simulink library "Hot_Water_Energy_Profile"  (R2018b)
settings: Solver=ode45  StartTime=0.0  StopTime=10.0  RelTol=1e-3  EnableMultiTasking=on
libraries: carnot x4
settings Model: Creator=lena.frank  LastModifiedBy=P41573
settings DataIOCC: LimitDataPoints=on  SaveFormat=Array  SignalLoggingSaveFormat=ModelDataLogs
settings OptimizationCC: ExpressionDepthLimit=2147483647  LifeSpan=inf
settings DebuggingCC: UnderspecifiedInitializationDetection=Classic  MergeDetectMultiDrivingBlocksExec=none  SolverPrmCheckMsg=warning  FcnCallInpInsideContextMsg=warning  StateNameClashWarn=warning  SFUnexpectedBacktrackingDiag=warning  SFNoUnconditionalDefaultTransitionDiag=warning  SFExecutionAtInitializationDiag=none
settings HardwareCC: ProdBitPerPointer=32  ProdBitPerSizeT=32  ProdBitPerPtrDiffT=32  ProdLargestAtomicFloat=None  ProdIntDivRoundTo=Undefined  ProdEndianess=Unspecified  ProdWordSize=32  ProdHWDeviceType=32-bit Generic
settings ModelReferenceCC: PropagateSignalLabelsOutOfModel=off
settings SFSimCC: SimUseLocalCustomCode=off
settings RTWCC: RTWUseLocalCustomCode=off
settings CodeAppCC: StateflowObjectComments=on
settings GRTTargetCC: TargetLangStandard=C89/C90 (ANSI)  GeneratePreprocessorConditionals=Disable all  CombineOutputUpdateFcns=off  GRTInterface=on
settings ConfigComp: CovMetricSettings=dw  CovHtmlReporting=on  CovSaveCumulativeToWorkspaceVar=on  CovSaveSingleToWorkspaceVar=on  CovExternalEMLEnable=off

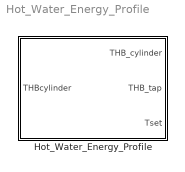
== system Hot_Water_Energy_Profile ==
  Hot_Water_Energy_Profile : Subsystem  mask(Hot Water Energy Profile){Tcw=10, mdot_nom=0.1, times=[7 12 19]*3600, energies=[4 2 4]*3600000, dT_set=[35 35 35], coeffs=[1 1 1]}
      mask prompts: Tcw "Cold water temperature in °C"; mdot_nom "Nominal massflow [kg/s]"; times "vector of start times [s]"; energies "vector of energies [J]"; dT_set "vector of temperature differences to the cold water [K]"; coeffs "vector of nominal massflow fractions [-]"
      mask help:
      | Domestic hot water consumption defined by an energy profile. This block uses the DHW_Energy_Tapping block.
      | The hot water of the cylinder entering the block is mixed with the cold water to reach the temperature setpoint. The necessary massflow through the cylinder is calculated by this block and set in the outport to the cylinder.
      mask Help: web(fullfile(path_carnot('help'),'HotWaterEnergyProfile.html'),'-helpbrowser')
      mask TypeOptions Tcw: T_cold_water_const/Value
      mask TypeOptions mdot_nom: DHW_Energy_Tapping/mdot_nom
      mask TypeOptions times: DHW_Energy_Tapping/times
      mask TypeOptions energies: DHW_Energy_Tapping/energies
      mask TypeOptions dT_set: DHW_Energy_Tapping/dT_set
      mask TypeOptions coeffs: DHW_Energy_Tapping/coeffs
      mask DialogControl Container3 Prompt: Profile of the water draw-offs
      mask Display:
      | text(15,120,'Energy-Profile')
      | plot(0,0,140,130,[70,76,78,63,65,70,70,10],[80,78,74,74,78,80,100,100],[23,23,20,10],[43,47,50,50],[10,10,20,28,30,10],[30,20,20,23,30,30],[22,17],[54,54],[20,20],[54,50],[90,90,50,50],[10,-0,-0,10],[63,64],[60,72],[61,62],[38,50],[60,61],[13,27],[90,85,81,76,70,65,59,54,50],[6,4,6,4,6,4,5,3,5],[68,69],[56,68],[68,68],[32,44],[67,67],[13,23],[73,73],[61,71],[73,73],[43,52],[74,73],[21,36],[78,77],[56,67],[79,79],[34,45],[78,77],[9,23],[82,81],[14,26])

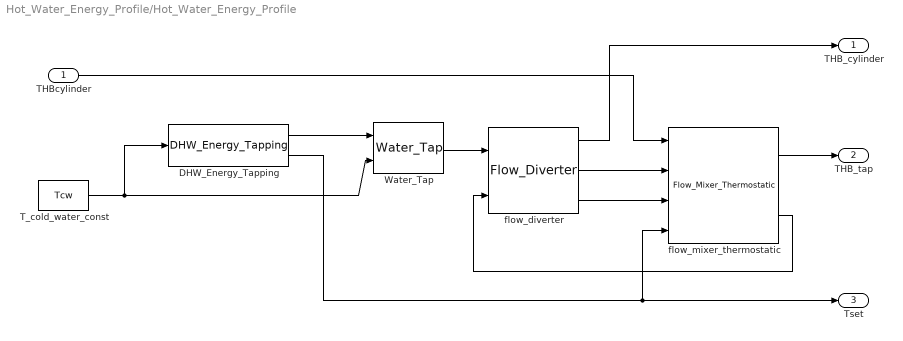
== system Hot_Water_Energy_Profile/Hot_Water_Energy_Profile ==
  THBcylinder : Inport
  DHW_Energy_Tapping : carnot/Load/Hot_Water_Tapping/DHW_Energy_Tapping  mdot_nom=mdot_nom  times=times  energies=energies  dT_set=dT_set  coeffs=coeffs
      settings: SourceProductName=Carnot
  T_cold_water_const : Constant  Value=Tcw
  Water_Tap : carnot/Load/Hot_Water_Tapping/Water_Tap  dia=0.02  p=2e5
      settings: SourceProductName=Carnot
  flow_diverter : carnot/Hydraulics/Flow_Diverter
      settings: SourceProductName=Carnot
  flow_mixer_thermostatic : carnot/Hydraulics/Flow_Mixer_Thermostatic  t=10
      settings: SourceProductName=Carnot
  THB_cylinder : Outport
  THB_tap : Outport  Port=2
  Tset : Outport  Port=3
  wires:
  flow_diverter/3 -> flow_mixer_thermostatic/3
  flow_diverter/2 -> flow_mixer_thermostatic/2
  flow_diverter/1 -> THB_cylinder/1
  THBcylinder/1 -> flow_mixer_thermostatic/1
  flow_mixer_thermostatic/1 -> THB_tap/1
  flow_mixer_thermostatic/2 -> flow_diverter/2
  Water_Tap/1 -> flow_diverter/1
  T_cold_water_const/1 -> DHW_Energy_Tapping/1, Water_Tap/2
  DHW_Energy_Tapping/1 -> Water_Tap/1
  DHW_Energy_Tapping/2 -> flow_mixer_thermostatic/4, Tset/1
